simulink model "Schemat"  (R2018a)
settings: Solver=ode45  StartTime=0.0  StopTime=czas  RelTol=1e-3
values from neighbouring files (symbols this model uses):
  cp = 1000    [Skrypt.m]
  Cv1 = cb*rob*Vw1    (= 49280000)    [Skrypt.m]
  Cv2 = cb*rob*Vw2    (= 55440000)    [Skrypt.m]
  czas_skoku = 50000    [Skrypt.m]
  dfk0 = fk * 0.12    (= 0.00659739402936)    [Skrypt.m]
  dTkz0 = 0    [Skrypt.m]
  dTzew0 = 0    [Skrypt.m]
  fk0 = fk *1.0    (= 0.054978283578)    [Skrypt.m]
  k0 = (1/3)*ks1    (= 5.27791522349)    [Skrypt.m]
  ks1 = (cp*rop*fk*(Tkzn-Tw1))/(Tw1-Tzewn+(1/3)*(Tw1-Tw2))    (= 15.8337456705)    [Skrypt.m]
  ks2 = ((1/3)*ks1*(Tw1-Tw2)+cp*rop*fk*(Tw1-Tw2))/(Tw2-Tzewn)    (= 10.1788365024)    [Skrypt.m]
  rop = 1.2    [Skrypt.m]
  Tkz0 = Tkzn * 1.0    (= 30)    [Skrypt.m]
  Tw10 = ((k0+cp*rop*fk0+ks2)*(cp*rop*fk0*Tkz0+ks1*Tzew0)+k0*ks2*Tzew0)/((cp*rop*fk0+ks1+k0)*(k0+cp*rop*fk0+ks2)-k0*(k0+cp*rop*fk0))    (= 20)    [Skrypt.m]
  Tw20 = (Tw10*(k0+cp*rop*fk0)+ks2*Tzew0)/(k0+cp*rop*fk0+ks2)    (= 15)    [Skrypt.m]
  Tzew0 = Tzewn + 0    (= -20)    [Skrypt.m]
settings Model: SnapshotBufferSize=1  SnapshotInterval=1  Creator=Mutungamiri  LastModifiedBy=Mutungamiri

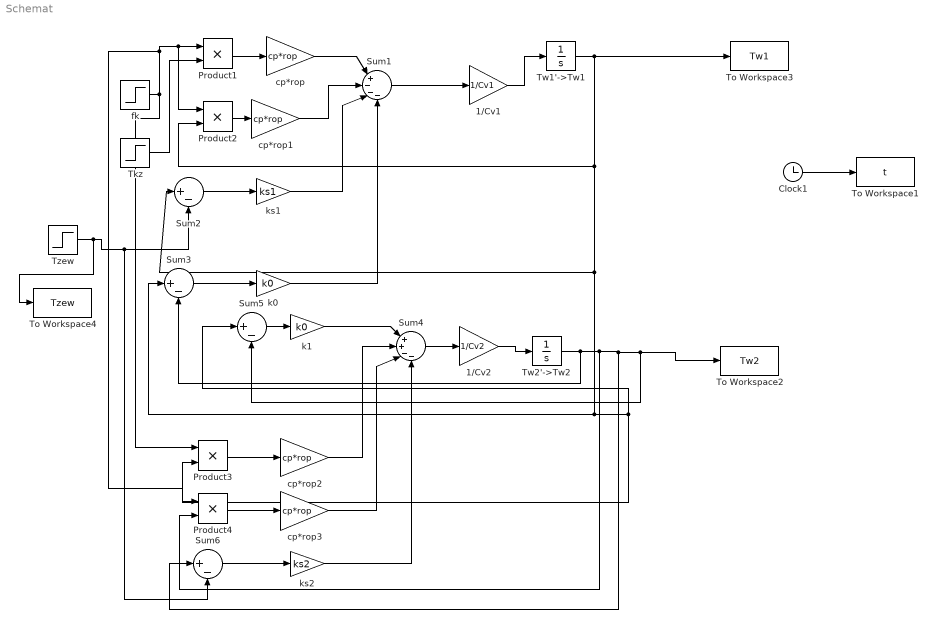
== system Schemat ==
  1/Cv1 : Gain  Gain=1/Cv1
  1/Cv2 : Gain  Gain=1/Cv2
  Clock1 : Clock
  Product{1..4} (4 alike) : Product
  Sum1 : Sum  Inputs=|+---
  Sum{2..3,5..6} (4 alike) : Sum  Inputs=|+-
  Sum4 : Sum  Inputs=|++--
  Tkz : Step  Time=czas_skoku  Before=Tkz0  After=Tkz0+dTkz0  SampleTime=0
  To Workspace1 : ToWorkspace  VariableName=t  SampleTime=-1
  To Workspace2 : ToWorkspace  VariableName=Tw2  SampleTime=-1
  To Workspace3 : ToWorkspace  VariableName=Tw1  SampleTime=-1
  To Workspace4 : ToWorkspace  VariableName=Tzew  SampleTime=-1
  Tw1'->Tw1 : Integrator  InitialCondition=Tw10
  Tw2'->Tw2 : Integrator  InitialCondition=Tw20
  Tzew : Step  Time=czas_skoku  Before=Tzew0  After=Tzew0+dTzew0  SampleTime=0
  cp*rop{,1..3} (4 alike) : Gain  Gain=cp*rop
  fk : Step  Time=czas_skoku  Before=fk0  After=fk0+dfk0  SampleTime=0
  k0 : Gain  Gain=k0
  k1 : Gain  Gain=k0
  ks1 : Gain  Gain=ks1
  ks2 : Gain  Gain=ks2
  wires:
  Clock1/1 -> To Workspace1/1
  1/Cv1/1 -> Tw1'->Tw1/1
  Sum1/1 -> 1/Cv1/1
  fk/1 -> Product2/1, Product1/1, Product4/1, Product3/1
  Tkz/1 -> Product1/2
  Product1/1 -> cp*rop/1
  cp*rop/1 -> Sum1/1
  cp*rop1/1 -> Sum1/2
  Product2/1 -> cp*rop1/1
  Tw1'->Tw1/1 -> To Workspace3/1, Sum5/1, Product3/2, Sum3/1, Sum2/1, Product2/2
  ks1/1 -> Sum1/3
  Sum2/1 -> ks1/1
  Tzew/1 -> To Workspace4/1, Sum6/2, Sum2/2
  k0/1 -> Sum1/4
  Sum3/1 -> k0/1
  Tw2'->Tw2/1 -> Product4/2, Sum6/1, To Workspace2/1, Sum5/2, Sum3/2
  1/Cv2/1 -> Tw2'->Tw2/1
  Sum4/1 -> 1/Cv2/1
  k1/1 -> Sum4/1
  Sum5/1 -> k1/1
  cp*rop2/1 -> Sum4/2
  Product3/1 -> cp*rop2/1
  cp*rop3/1 -> Sum4/3
  Product4/1 -> cp*rop3/1
  ks2/1 -> Sum4/4
  Sum6/1 -> ks2/1
